simulink model "testtest"  (Simulink 7.6)
settings: Solver=ode45  StartTime=0.0  StopTime=100  RelTol=1e-3
settings Model: Creator=Administrator  LastModifiedBy=Administrator
settings DebuggingCC: AlgebraicLoopMsg=none  ArtificialAlgebraicLoopMsg=none  SolverPrmCheckMsg=none  UnknownTsInhSupMsg=none

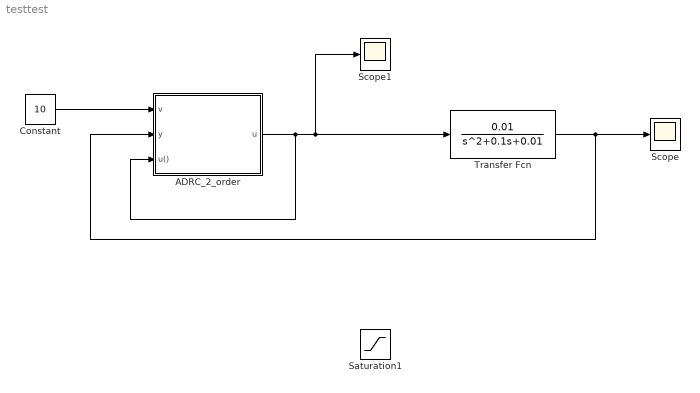
== system testtest ==
  ADRC_2_order : Subsystem  AncestorBlock=ADRC/ADRC/ADRC_2rd/ADRC_2_order  mask{h=0.1, TD=[0.1,0.1], ESO=[10,30,25,0.1], NLSEF=[0.1,2,0.2], b0=1}
      mask prompts: h "h="; TD "TD[r0,h]="; ESO "ESO[B01,B02,B03,D]="; NLSEF "NLSEF[c,r1,h1]="; b0 "b0="
  Constant : Constant  Value=10
  Saturation1 : Saturate  UpperLimit=100  LowerLimit=0
  Scope : Scope
      settings: YMin=5.25  YMax=10.25  DataFormat=Array
  Scope1 : Scope
      settings: TimeRange=50  YMin=0  YMax=250  DataFormat=Array
  Transfer Fcn : TransferFcn  Numerator=0.01  Denominator=[1 0.1 0.01]
  wires:
  Constant/1 -> ADRC_2_order/1(v)
  ADRC_2_order/1(u) -> ADRC_2_order/3(u()), Scope1/1, Transfer Fcn/1
  Transfer Fcn/1 -> Scope/1, ADRC_2_order/2(y)

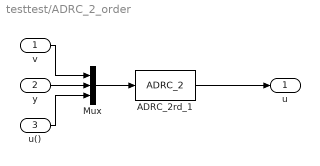
== system testtest/ADRC_2_order ==
  v : Inport
  y : Inport  Port=2
  u() : Inport  Port=3
  ADRC_2rd_1 : S-Function  FunctionName=ADRC_2  Parameters=h,TD,ESO,NLSEF,b0  EnableBusSupport=off
  Mux : Mux  Inputs=3
  u : Outport
  wires:
  u()/1 -> Mux/3
  Mux/1 -> ADRC_2rd_1/1
  y/1 -> Mux/2
  v/1 -> Mux/1
  ADRC_2rd_1/1 -> u/1
